simulink model "calculate_k13"  (R2022b)
settings: Solver=VariableStepAuto  StartTime=0.0  StopTime=10.0  RelTol=1e-3
values from neighbouring files (symbols this model uses):
  k3 = -0.0006    [run_first.m]
settings Model: Creator=fabian  LastModifiedBy=fabian

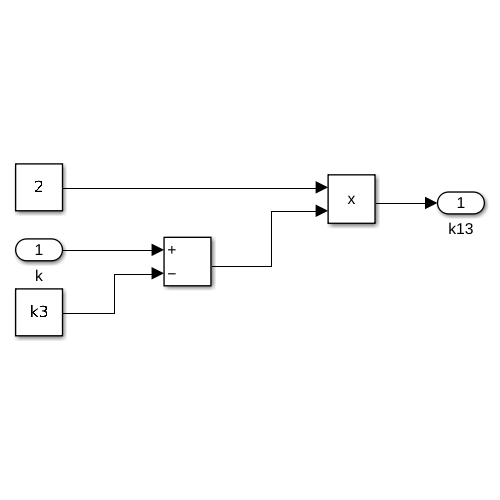
[thumbnail: Simulink's stored preview of the top-level diagram]
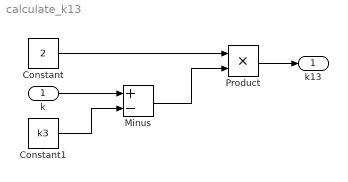
== system calculate_k13 ==
  k : Inport
  Constant : Constant  Value=2
  Constant1 : Constant  Value=k3
  Minus : Sum  Inputs=+-
  Product : Product
  k13 : Outport
  wires:
  Minus/1 -> Product/2
  Constant/1 -> Product/1
  Constant1/1 -> Minus/2
  Product/1 -> k13/1
  k/1 -> Minus/1
